simulink model "Control_test"  (R2014b)
settings: Solver=FixedStepDiscrete  StartTime=0.0  StopTime=Inf  FixedStep=0.001  RelTol=1e-3
PostLoadFcn:
  | , if any(exist('dsrtsu_mdlpostloadfcn', 'file') == [2, 3, 6]), try dsrtsu_mdlpostloadfcn('Execute', bdroot); catch fprintf('Error in PostLoadFcn (dsrtsu_mdlpostloadfcn) for model "%s":\n %s\n', bdroot, lasterr); end, end,
undefined symbols (not defined in the file or in its folder): dtLocal, slcm
libraries: rtican x163, simulink x14
(part 10 of 34)

== system Control_test/InputProcessing/CameraCanProcessing/Obstacle_Data_A_4 ==
  Bus Creator : BusCreator  Inputs=11
  Obstacle_Data_A_4 : rtican/RTICAN Receive (RX)   Reserved1=[]  Reserved2=[]  Reserved3=[]  Reserved4=[]  SfcnMessage=[]  Msg_Struct=[]  BoardTypeNo=[]  BoardNo=[]  ChannelNo=[]  Parameters=[]  DialogFcn=[]  UnitName=[]  Revision=[]  UnitValues=[]  DSProperties=struct('RTI',struct('Version',uint32(5),'BlockType',struct('isSLSource',uint8(1),'isSLSink',uint8(1),'isHWSource',uint8(0),'isHWSink',uint8(0),'isSetup',uint8(0),'isInline',uint8(1),'isNonInline',uint8(0),'isInterrupt',uint8(0),'isChannelwise',uint8(0)),'IOBoardType','RTICAN','UnitType','MESSAGE','Identifier','RX','DialogType','MSVC','BlockSet','RTICAN','SlaveProcessor','CAN'))  RTIBlockInterface=struct('OutputPortsWidth',int32([1 1 1 1 1 1 1 1 1 1 1]),'OutputPortsActive',[1 1 1 1 1 1 1 1 1 1 1],'OutputPortsName',{{'Alive_Counter_A_4','ObjectIdentifier_A_4','ObjectAge_A_4','AngleRate_A_4','AngleLeft_A_4','AngleRight_A_4','MotionStatus_A_4','ObjectLane_A_4','CIPV_A_4','ObstacleBrakeLights_A_4','BlinkerInfo_A_4'}},'OutputPortsDataType',{{'SS_DOUBLE','SS_DOUBLE','SS_DOUBLE','SS_DOUBLE','SS_DOUBLE','SS_DOUBLE','SS_DOUBLE','SS_DOUBLE','SS_DOUBLE','SS_DOUBLE','SS_DOUBLE'}},'OutputPortsLabel',{{'Alive_Counter_A_4','ObjectIdentifier_A_4','ObjectAge_A_4','AngleRate_A_4','AngleLeft_A_4','AngleRight_A_4','MotionStatus_A_4','ObjectLane_A_4','CIPV_A_4','ObstacleBrakeLights_A_4','BlinkerInfo_A_4'}},'OutputPortsLabelMode','ON','InputPortsWidth',int32(0),'InputPortsActive',0,'DialogFcn','rtican_message_interface_gui','BlockDisplay',{{'','center'}},'IconTransparency','on','ParameterTunableNames',{{}},'InitLevel',3,'BlockName',struct('Token',{{'Obstacle_Data_A_4'}}),'SampleTime',{{0.01}},'TriggerPort',{{'none'}},'EnablePort',{{'none'}})  RTIBlockParameters=struct('BoardTypeNo',{{1,'OFF',[]}},'BoardNo',{{1,'ON',[1 16]}},'ChannelNo',{{2,'ON',[1 2]}},'Parameters',{{struct('DataFileSupport',struct('DataFileSelectedMaster',1,'DataFileSelectedLocal',0,'DataFileName',['c:\users\mpc\dropbox\cpg_test_2014\t4_rfs_demo\hyundai car setup\rt2000_can_mod.dbc|c:\users\mpc\dropbox\cpg_test_2014\t4_rfs_demo\hyundai car setup\mobileye spec new\mobileye_mando_camera_ucb_v2.dbc|'],'DataFileDate',{{{['13-Nov-2012 16:29:35']},{['18-Sep-2013 10:55:24']}}},'SelectedFile',['<no file selected>'],'InterfaceFcn','rtican_dbc_file_parser'),'Options',struct('StatusSelected',0,'TimeSelected',0,'DeltaTimeSelected',0,'BytePortSelected',0,'MessageLengthSelected',0,'TriggerPort',struct('Selected',0,'TriggerType',0),'UserCoding',struct('Selected',0,'InterfaceFile','UserDecodingFile','FcnName','UserDecodeFcn','InportSelected',0,'InportWidth',1,'OutportSelected',0,'OutportWidth',1),'EnablePortSelected',0,'SignalOnPortnameSelected',1,'UseRXService',0),'Message',struct('MsgOnBlocknameSelected',1,'MsgName','Obstacle_Data_A_4','MsgIdFormat',0,'MsgId',1858,'MsgLength',8,'NumSignals',11,'SampleTime',0.01,'Signal',struct('SgnName',{'Alive_Counter_A_4','ObjectIdentifier_A_4','ObjectAge_A_4','AngleRate_A_4','AngleLeft_A_4','AngleRight_A_4','MotionStatus_A_4','ObjectLane_A_4','CIPV_A_4','ObstacleBrakeLights_A_4','BlinkerInfo_A_4'},'SgnStartBit',{0,2,8,16,28,40,52,56,60,61,62},'SgnLength',{2,6,8,12,12,12,4,4,1,1,2},'SgnType',{0,0,0,0,0,0,0,0,0,0,0},'ModeValue',{-1,-1,-1,-1,-1,-1,-1,-1,-1,-1,-1},'DataType',{0,0,0,0,0,0,0,0,0,0,0},'ByteLayout',{0,0,0,0,0,0,0,0,0,0,0},'Factor',{1,1,1,0.05,0.05,0.05,1,1,1,1,1},'Offset',{0,0,0,-100,-100,-100,0,0,0,0,0},'SgnComment',{{''},{''},{''},{''},{''},{''},{''},{''},{''},{''},{''}},'SgnUnit',{'','','','Deg','Deg','Deg','','','','',''},'Min',{0,0,0,0,0,0,0,0,0,0,0},'Max',{0,0,0,0,0,0,0,0,0,0,0},'SLDataType',{'SS_DOUBLE','SS_DOUBLE','SS_DOUBLE','SS_DOUBLE','SS_DOUBLE','SS_DOUBLE','SS_DOUBLE','SS_DOUBLE','SS_DOUBLE','SS_DOUBLE','SS_DOUBLE'}),'MsgIdNumFormat',1,'MsgComment',{{''}}),'Version',1.2,'general',struct('isFromLib',0)),'OFF',[]}},'GroupId',{{struct('Group',{{'RTICAN'}},'No',2,'Behavior',{{'NAMECHANGE'}},'BlockType',{{'SINK'}},'NameChangeFlag',0),'OFF',[]}},'SFcnRTICANMessage',{{struct('MsgType','RX','SFcnPortType','Scalar','MsgName','Obstacle_Data_A_4','MsgIdFormat','STD','MsgId',1858,'MsgLength',8,'NumSignals',11,'SampleTime',0.01,'Signal',struct('SgnName',{'Alive_Counter_A_4','ObjectIdentifier_A_4','ObjectAge_A_4','AngleRate_A_4','AngleLeft_A_4','AngleRight_A_4','MotionStatus_A_4','ObjectLane_A_4','CIPV_A_4','ObstacleBrakeLights_A_4','BlinkerInfo_A_4'},'SgnStartBit',{0,2,8,16,28,40,52,56,60,61,62},'SgnLength',{2,6,8,12,12,12,4,4,1,1,2},'SgnType',{'standard','standard','standard','standard','standard','standard','standard','standard','standard','standard','standard'},'ModeValue',{-1,-1,-1,-1,-1,-1,-1,-1,-1,-1,-1},'DataType',{['unsigned int'],['unsigned int'],['unsigned int'],['unsigned int'],['unsigned int'],['unsigned int'],['unsigned int'],['unsigned int'],['unsigned int'],['unsigned int'],['unsigned int']},'ByteLayout',{['little endian'],['little endian'],['little endian'],['little endian'],['little endian'],['little endian'],['little endian'],['little endian'],['little endian'],['little endian'],['little endian']},'Factor',{1,1,1,0.05,0.05,0.05,1,1,1,1,1},'Offset',{0,0,0,-100,-100,-100,0,0,0,0,0},'SLDataType',{'SS_DOUBLE','SS_DOUBLE','SS_DOUBLE','SS_DOUBLE','SS_DOUBLE','SS_DOUBLE','SS_DOUBLE','SS_DOUBLE','SS_DOUBLE','SS_DOUBLE','SS_DOUBLE'}),'StatusSelected','no','TimeSelected','no','DeltaTimeSelected','no','BytePortSelected','no','MessageLengthSelected','no','TriggerPort',struct('Selected','no','TriggerType',0),'UserCoding',struct('Selected','no','InterfaceFile','UserDecodingFile','FcnName','UserDecodeFcn','InportSelected','no','InportWidth',1,'OutportSelected','no','OutportWidth',1),'EnablePortSelected','no','UseRXService','no','BoardType','DS1','BoardNo',1,'ControllerNo',2),'OFF',[]}},'TLCFileName',{{'rtican_rx_message','OFF',[]}})  RTISFcnParameters=struct('SFcnRTICANMessage','struct','TLCFileName','char')  RTIBlockParaDefault=struct('BoardTypeNo',4302,'BoardNo',1,'ChannelNo',1,'Parameters',struct('DataFileSupport',struct('DataFileSelectedMaster',0,'DataFileSelectedLocal',0,'DataFileName','','DataFileDate','','SelectedFile',['<no file selected>']),'Options',struct('StatusSelected',1,'TimeSelected',1,'DeltaTimeSelected',1,'BytePortSelected',0,'MessageLengthSelected',0,'TriggerPort',struct('Selected',0,'TriggerType','rising'),'UserCoding',struct('Selected',0,'InterfaceFile','UserDecodingFile','FcnName','UserDecodeFcn','InportSelected',0,'InportWidth',1,'OutportSelected',0,'OutportWidth',1),'EnablePortSelected',0,'SignalOnPortnameSelected',1,'UseRXService',0),'Message',struct('MsgOnBlocknameSelected',0,'MsgName',['RX Message'],'MsgIdFormat',0,'MsgId',100,'MsgLength',8,'NumSignals',1,'SampleTime',-1,'Signal',struct('SgnName',['RX signal'],'SgnStartBit',0,'SgnLength',8,'SgnType',0,'ModeValue',-1,'DataType',0,'SLDataType','SS_DOUBLE','ByteLayout',0,'Factor',1,'Offset',0,'Min',0,'Max',255,'SgnComment',{{}},'SgnUnit',''),'MsgIdNumFormat',0,'MsgComment',{{''}}),'Version',1.2,'general',struct('isFromLib',1)),'GroupId',struct('Group',{{'RTICAN'}},'No',1,'Behavior',{{'NAMECHANGE'}},'BlockType',{{'SINK'}},'NameChangeFlag',0),'SFcnRTICANMessage',struct('MsgType','RX','MsgName',['RX Message'],'MsgIdFormat','STD','MsgId',100,'MsgLength',8,'NumSignals',1,'SampleTime',-1,'Signal',struct('SgnName',['RX signal'],'SgnStartBit',0,'SgnLength',8,'SgnType','standard','ModeValue',-1,'DataType',['unsigned int'],'ByteLayout',['little endian'],'SLDataType','SS_DOUBLE','Factor',1,'Offset',0),'StatusSelected','yes','TimeSelected','yes','DeltaTimeSelected','yes','BytePortSelected','no','MessageLengthSelected','no','EnablePortSelected','no','UserCoding',struct('Selected','no','InterfaceFile','UserDecodingFile','FcnName','UserDecodeFcn','InportSelected','no','InportWidth',1,'OutportSelected','no','OutportWidth',1),'TriggerPort',struct('Selected','no','TriggerType','rising'),'UseRXService','no','BoardType','DS4302','BoardNo',1,'ControllerNo',1,'SFcnPortType','Scalar'),'TLCFileName','rtican_rx_message')
      settings: AttributesFormatString=Group Id: RTICAN2\n
  Obstacle_Data_A_4_CAN : Outport
  wires:
  Bus Creator/1 -> Obstacle_Data_A_4_CAN/1
  Obstacle_Data_A_4/1 -> Bus Creator/1  "Alive_Counter_A_4"
  Obstacle_Data_A_4/2 -> Bus Creator/2  "ObjectIdentifier_A_4"
  Obstacle_Data_A_4/3 -> Bus Creator/3  "ObjectAge_A_4"
  Obstacle_Data_A_4/4 -> Bus Creator/4  "AngleRate_A_4"
  Obstacle_Data_A_4/5 -> Bus Creator/5  "AngleLeft_A_4"
  Obstacle_Data_A_4/6 -> Bus Creator/6  "AngleRight_A_4"
  Obstacle_Data_A_4/7 -> Bus Creator/7  "MotionStatus_A_4"
  Obstacle_Data_A_4/8 -> Bus Creator/8  "ObjectLane_A_4"
  Obstacle_Data_A_4/9 -> Bus Creator/9  "CIPV_A_4"
  Obstacle_Data_A_4/10 -> Bus Creator/10  "ObstacleBrakeLights_A_4"
  Obstacle_Data_A_4/11 -> Bus Creator/11  "BlinkerInfo_A_4"

== system Control_test/InputProcessing/CameraCanProcessing/Obstacle_Data_A_5 ==
  Bus Creator : BusCreator  Inputs=11
  Obstacle_Data_A_5 : rtican/RTICAN Receive (RX)   Reserved1=[]  Reserved2=[]  Reserved3=[]  Reserved4=[]  SfcnMessage=[]  Msg_Struct=[]  BoardTypeNo=[]  BoardNo=[]  ChannelNo=[]  Parameters=[]  DialogFcn=[]  UnitName=[]  Revision=[]  UnitValues=[]  DSProperties=struct('RTI',struct('Version',uint32(5),'BlockType',struct('isSLSource',uint8(1),'isSLSink',uint8(1),'isHWSource',uint8(0),'isHWSink',uint8(0),'isSetup',uint8(0),'isInline',uint8(1),'isNonInline',uint8(0),'isInterrupt',uint8(0),'isChannelwise',uint8(0)),'IOBoardType','RTICAN','UnitType','MESSAGE','Identifier','RX','DialogType','MSVC','BlockSet','RTICAN','SlaveProcessor','CAN'))  RTIBlockInterface=struct('OutputPortsWidth',int32([1 1 1 1 1 1 1 1 1 1 1]),'OutputPortsActive',[1 1 1 1 1 1 1 1 1 1 1],'OutputPortsName',{{'Alive_Counter_A_5','ObjectIdentifier_A_5','ObjectAge_A_5','AngleRate_A_5','AngleLeft_A_5','AngleRight_A_5','MotionStatus_A_5','ObjectLane_A_5','CIPV_A_5','ObstacleBrakeLights_A_5','BlinkerInfo_A_5'}},'OutputPortsDataType',{{'SS_DOUBLE','SS_DOUBLE','SS_DOUBLE','SS_DOUBLE','SS_DOUBLE','SS_DOUBLE','SS_DOUBLE','SS_DOUBLE','SS_DOUBLE','SS_DOUBLE','SS_DOUBLE'}},'OutputPortsLabel',{{'Alive_Counter_A_5','ObjectIdentifier_A_5','ObjectAge_A_5','AngleRate_A_5','AngleLeft_A_5','AngleRight_A_5','MotionStatus_A_5','ObjectLane_A_5','CIPV_A_5','ObstacleBrakeLights_A_5','BlinkerInfo_A_5'}},'OutputPortsLabelMode','ON','InputPortsWidth',int32(0),'InputPortsActive',0,'DialogFcn','rtican_message_interface_gui','BlockDisplay',{{'','center'}},'IconTransparency','on','ParameterTunableNames',{{}},'InitLevel',3,'BlockName',struct('Token',{{'Obstacle_Data_A_5'}}),'SampleTime',{{0.01}},'TriggerPort',{{'none'}},'EnablePort',{{'none'}})  RTIBlockParameters=struct('BoardTypeNo',{{1,'OFF',[]}},'BoardNo',{{1,'ON',[1 16]}},'ChannelNo',{{2,'ON',[1 2]}},'Parameters',{{struct('DataFileSupport',struct('DataFileSelectedMaster',1,'DataFileSelectedLocal',1,'DataFileName',['c:\users\mpc\desktop\hyundai car setup\rt2000_can_mod.dbc|c:\users\mpc\desktop\hyundai car setup\mobileye spec new\mobileye_mando_camera_ucb_v2.dbc|'],'DataFileDate',['18-Sep-2013 17:55:24'],'SelectedFile','..\..\dbcfiles\mobileye_mando_camera_ucb_v2.dbc','InterfaceFcn','rtican_dbc_file_parser'),'Options',struct('StatusSelected',0,'TimeSelected',0,'DeltaTimeSelected',0,'BytePortSelected',0,'MessageLengthSelected',0,'TriggerPort',struct('Selected',0,'TriggerType',0),'UserCoding',struct('Selected',0,'InterfaceFile','UserDecodingFile','FcnName','UserDecodeFcn','InportSelected',0,'InportWidth',1,'OutportSelected',0,'OutportWidth',1),'EnablePortSelected',0,'SignalOnPortnameSelected',1,'UseRXService',0),'Message',struct('MsgOnBlocknameSelected',1,'MsgName','Obstacle_Data_A_5','MsgIdFormat',0,'MsgId',1861,'MsgLength',8,'NumSignals',11,'SampleTime',0.01,'Signal',struct('SgnName',{'Alive_Counter_A_5','ObjectIdentifier_A_5','ObjectAge_A_5','AngleRate_A_5','AngleLeft_A_5','AngleRight_A_5','MotionStatus_A_5','ObjectLane_A_5','CIPV_A_5','ObstacleBrakeLights_A_5','BlinkerInfo_A_5'},'SgnStartBit',{0,2,8,16,28,40,52,56,60,61,62},'SgnLength',{2,6,8,12,12,12,4,4,1,1,2},'ByteLayout',{0,0,0,0,0,0,0,0,0,0,0},'Factor',{1,1,1,0.05,0.05,0.05,1,1,1,1,1},'Offset',{0,0,0,-100,-100,-100,0,0,0,0,0},'SgnComment',{'','','','','','','','','','',''},'SgnUnit',{'','','','Deg','Deg','Deg','','','','',''},'Min',{0,0,0,0,0,0,0,0,0,0,0},'Max',{0,0,0,0,0,0,0,0,0,0,0},'SgnType',{0,0,0,0,0,0,0,0,0,0,0},'SLDataType',{'SS_DOUBLE','SS_DOUBLE','SS_DOUBLE','SS_DOUBLE','SS_DOUBLE','SS_DOUBLE','SS_DOUBLE','SS_DOUBLE','SS_DOUBLE','SS_DOUBLE','SS_DOUBLE'},'DataType',{0,0,0,0,0,0,0,0,0,0,0},'ModeValue',{-1,-1,-1,-1,-1,-1,-1,-1,-1,-1,-1}),'MsgIdNumFormat',0,'MsgComment',{{''}}),'Version',1.2,'general',struct('isFromLib',0)),'OFF',[]}},'GroupId',{{struct('Group',{{'RTICAN'}},'No',2,'Behavior',{{'NAMECHANGE'}},'BlockType',{{'SINK'}},'NameChangeFlag',0),'OFF',[]}},'SFcnRTICANMessage',{{struct('MsgType','RX','SFcnPortType','Scalar','MsgName','Obstacle_Data_A_5','MsgIdFormat','STD','MsgId',1861,'MsgLength',8,'NumSignals',11,'SampleTime',0.01,'Signal',struct('SgnName',{'Alive_Counter_A_5','ObjectIdentifier_A_5','ObjectAge_A_5','AngleRate_A_5','AngleLeft_A_5','AngleRight_A_5','MotionStatus_A_5','ObjectLane_A_5','CIPV_A_5','ObstacleBrakeLights_A_5','BlinkerInfo_A_5'},'SgnStartBit',{0,2,8,16,28,40,52,56,60,61,62},'SgnLength',{2,6,8,12,12,12,4,4,1,1,2},'ByteLayout',{['little endian'],['little endian'],['little endian'],['little endian'],['little endian'],['little endian'],['little endian'],['little endian'],['little endian'],['little endian'],['little endian']},'Factor',{1,1,1,0.05,0.05,0.05,1,1,1,1,1},'Offset',{0,0,0,-100,-100,-100,0,0,0,0,0},'SgnType',{'standard','standard','standard','standard','standard','standard','standard','standard','standard','standard','standard'},'SLDataType',{'SS_DOUBLE','SS_DOUBLE','SS_DOUBLE','SS_DOUBLE','SS_DOUBLE','SS_DOUBLE','SS_DOUBLE','SS_DOUBLE','SS_DOUBLE','SS_DOUBLE','SS_DOUBLE'},'DataType',{['unsigned int'],['unsigned int'],['unsigned int'],['unsigned int'],['unsigned int'],['unsigned int'],['unsigned int'],['unsigned int'],['unsigned int'],['unsigned int'],['unsigned int']},'ModeValue',{-1,-1,-1,-1,-1,-1,-1,-1,-1,-1,-1}),'StatusSelected','no','TimeSelected','no','DeltaTimeSelected','no','BytePortSelected','no','MessageLengthSelected','no','TriggerPort',struct('Selected','no','TriggerType',0),'UserCoding',struct('Selected','no','InterfaceFile','UserDecodingFile','FcnName','UserDecodeFcn','InportSelected','no','InportWidth',1,'OutportSelected','no','OutportWidth',1),'EnablePortSelected','no','UseRXService','no','BoardType','DS1','BoardNo',1,'ControllerNo',2),'OFF',[]}},'TLCFileName',{{'rtican_rx_message','OFF',[]}})  RTISFcnParameters=struct('SFcnRTICANMessage','struct','TLCFileName','char')  RTIBlockParaDefault=struct('BoardTypeNo',4302,'BoardNo',1,'ChannelNo',1,'Parameters',struct('DataFileSupport',struct('DataFileSelectedMaster',0,'DataFileSelectedLocal',0,'DataFileName','','DataFileDate','','SelectedFile',['<no file selected>']),'Options',struct('StatusSelected',1,'TimeSelected',1,'DeltaTimeSelected',1,'BytePortSelected',0,'MessageLengthSelected',0,'TriggerPort',struct('Selected',0,'TriggerType','rising'),'UserCoding',struct('Selected',0,'InterfaceFile','UserDecodingFile','FcnName','UserDecodeFcn','InportSelected',0,'InportWidth',1,'OutportSelected',0,'OutportWidth',1),'EnablePortSelected',0,'SignalOnPortnameSelected',1,'UseRXService',0),'Message',struct('MsgOnBlocknameSelected',0,'MsgName',['RX Message'],'MsgIdFormat',0,'MsgId',100,'MsgLength',8,'NumSignals',1,'SampleTime',-1,'Signal',struct('SgnName',['RX signal'],'SgnStartBit',0,'SgnLength',8,'SgnType',0,'ModeValue',-1,'DataType',0,'SLDataType','SS_DOUBLE','ByteLayout',0,'Factor',1,'Offset',0,'Min',0,'Max',255,'SgnComment',{{}},'SgnUnit',''),'MsgIdNumFormat',0,'MsgComment',{{''}}),'Version',1.2,'general',struct('isFromLib',1)),'GroupId',struct('Group',{{'RTICAN'}},'No',1,'Behavior',{{'NAMECHANGE'}},'BlockType',{{'SINK'}},'NameChangeFlag',0),'SFcnRTICANMessage',struct('MsgType','RX','MsgName',['RX Message'],'MsgIdFormat','STD','MsgId',100,'MsgLength',8,'NumSignals',1,'SampleTime',-1,'Signal',struct('SgnName',['RX signal'],'SgnStartBit',0,'SgnLength',8,'SgnType','standard','ModeValue',-1,'DataType',['unsigned int'],'ByteLayout',['little endian'],'SLDataType','SS_DOUBLE','Factor',1,'Offset',0),'StatusSelected','yes','TimeSelected','yes','DeltaTimeSelected','yes','BytePortSelected','no','MessageLengthSelected','no','EnablePortSelected','no','UserCoding',struct('Selected','no','InterfaceFile','UserDecodingFile','FcnName','UserDecodeFcn','InportSelected','no','InportWidth',1,'OutportSelected','no','OutportWidth',1),'TriggerPort',struct('Selected','no','TriggerType','rising'),'UseRXService','no','BoardType','DS4302','BoardNo',1,'ControllerNo',1,'SFcnPortType','Scalar'),'TLCFileName','rtican_rx_message')
      settings: AttributesFormatString=Group Id: RTICAN2\n
  Obstacle_Data_A_5_CAN : Outport
  wires:
  Bus Creator/1 -> Obstacle_Data_A_5_CAN/1
  Obstacle_Data_A_5/1 -> Bus Creator/1  "Alive_Counter_A_5"
  Obstacle_Data_A_5/2 -> Bus Creator/2  "ObjectIdentifier_A_5"
  Obstacle_Data_A_5/3 -> Bus Creator/3  "ObjectAge_A_5"
  Obstacle_Data_A_5/4 -> Bus Creator/4  "AngleRate_A_5"
  Obstacle_Data_A_5/5 -> Bus Creator/5  "AngleLeft_A_5"
  Obstacle_Data_A_5/6 -> Bus Creator/6  "AngleRight_A_5"
  Obstacle_Data_A_5/7 -> Bus Creator/7  "MotionStatus_A_5"
  Obstacle_Data_A_5/8 -> Bus Creator/8  "ObjectLane_A_5"
  Obstacle_Data_A_5/9 -> Bus Creator/9  "CIPV_A_5"
  Obstacle_Data_A_5/10 -> Bus Creator/10  "ObstacleBrakeLights_A_5"
  Obstacle_Data_A_5/11 -> Bus Creator/11  "BlinkerInfo_A_5"

== system Control_test/InputProcessing/CameraCanProcessing/Obstacle_Data_A_6 ==
  Bus Creator : BusCreator  Inputs=11
  Obstacle_Data_A_6 : rtican/RTICAN Receive (RX)   Reserved1=[]  Reserved2=[]  Reserved3=[]  Reserved4=[]  SfcnMessage=[]  Msg_Struct=[]  BoardTypeNo=[]  BoardNo=[]  ChannelNo=[]  Parameters=[]  DialogFcn=[]  UnitName=[]  Revision=[]  UnitValues=[]  DSProperties=struct('RTI',struct('Version',uint32(5),'BlockType',struct('isSLSource',uint8(1),'isSLSink',uint8(1),'isHWSource',uint8(0),'isHWSink',uint8(0),'isSetup',uint8(0),'isInline',uint8(1),'isNonInline',uint8(0),'isInterrupt',uint8(0),'isChannelwise',uint8(0)),'IOBoardType','RTICAN','UnitType','MESSAGE','Identifier','RX','DialogType','MSVC','BlockSet','RTICAN','SlaveProcessor','CAN'))  RTIBlockInterface=struct('OutputPortsWidth',int32([1 1 1 1 1 1 1 1 1 1 1]),'OutputPortsActive',[1 1 1 1 1 1 1 1 1 1 1],'OutputPortsName',{{'Alive_Counter_A_6','ObjectIdentifier_A_6','ObjectAge_A_6','AngleRate_A_6','AngleLeft_A_6','AngleRight_A_6','MotionStatus_A_6','ObjectLane_A_6','CIPV_A_6','ObstacleBrakeLights_A_6','BlinkerInfo_A_6'}},'OutputPortsDataType',{{'SS_DOUBLE','SS_DOUBLE','SS_DOUBLE','SS_DOUBLE','SS_DOUBLE','SS_DOUBLE','SS_DOUBLE','SS_DOUBLE','SS_DOUBLE','SS_DOUBLE','SS_DOUBLE'}},'OutputPortsLabel',{{'Alive_Counter_A_6','ObjectIdentifier_A_6','ObjectAge_A_6','AngleRate_A_6','AngleLeft_A_6','AngleRight_A_6','MotionStatus_A_6','ObjectLane_A_6','CIPV_A_6','ObstacleBrakeLights_A_6','BlinkerInfo_A_6'}},'OutputPortsLabelMode','ON','InputPortsWidth',int32(0),'InputPortsActive',0,'DialogFcn','rtican_message_interface_gui','BlockDisplay',{{'','center'}},'IconTransparency','on','ParameterTunableNames',{{}},'InitLevel',3,'BlockName',struct('Token',{{'Obstacle_Data_A_6'}}),'SampleTime',{{0.01}},'TriggerPort',{{'none'}},'EnablePort',{{'none'}})  RTIBlockParameters=struct('BoardTypeNo',{{1,'OFF',[]}},'BoardNo',{{1,'ON',[1 16]}},'ChannelNo',{{2,'ON',[1 2]}},'Parameters',{{struct('DataFileSupport',struct('DataFileSelectedMaster',1,'DataFileSelectedLocal',1,'DataFileName',['c:\users\mpc\desktop\hyundai car setup\rt2000_can_mod.dbc|c:\users\mpc\desktop\hyundai car setup\mobileye spec new\mobileye_mando_camera_ucb_v2.dbc|'],'DataFileDate',['18-Sep-2013 17:55:24'],'SelectedFile','..\..\dbcfiles\mobileye_mando_camera_ucb_v2.dbc','InterfaceFcn','rtican_dbc_file_parser'),'Options',struct('StatusSelected',0,'TimeSelected',0,'DeltaTimeSelected',0,'BytePortSelected',0,'MessageLengthSelected',0,'TriggerPort',struct('Selected',0,'TriggerType',0),'UserCoding',struct('Selected',0,'InterfaceFile','UserDecodingFile','FcnName','UserDecodeFcn','InportSelected',0,'InportWidth',1,'OutportSelected',0,'OutportWidth',1),'EnablePortSelected',0,'SignalOnPortnameSelected',1,'UseRXService',0),'Message',struct('MsgOnBlocknameSelected',1,'MsgName','Obstacle_Data_A_6','MsgIdFormat',0,'MsgId',1864,'MsgLength',8,'NumSignals',11,'SampleTime',0.01,'Signal',struct('SgnName',{'Alive_Counter_A_6','ObjectIdentifier_A_6','ObjectAge_A_6','AngleRate_A_6','AngleLeft_A_6','AngleRight_A_6','MotionStatus_A_6','ObjectLane_A_6','CIPV_A_6','ObstacleBrakeLights_A_6','BlinkerInfo_A_6'},'SgnStartBit',{0,2,8,16,28,40,52,56,60,61,62},'SgnLength',{2,6,8,12,12,12,4,4,1,1,2},'ByteLayout',{0,0,0,0,0,0,0,0,0,0,0},'Factor',{1,1,1,0.05,0.05,0.05,1,1,1,1,1},'Offset',{0,0,0,-100,-100,-100,0,0,0,0,0},'SgnComment',{'','','','','','','','','','',''},'SgnUnit',{'','','','Deg','Deg','Deg','','','','',''},'Min',{0,0,0,0,0,0,0,0,0,0,0},'Max',{0,0,0,0,0,0,0,0,0,0,0},'SgnType',{0,0,0,0,0,0,0,0,0,0,0},'SLDataType',{'SS_DOUBLE','SS_DOUBLE','SS_DOUBLE','SS_DOUBLE','SS_DOUBLE','SS_DOUBLE','SS_DOUBLE','SS_DOUBLE','SS_DOUBLE','SS_DOUBLE','SS_DOUBLE'},'DataType',{0,0,0,0,0,0,0,0,0,0,0},'ModeValue',{-1,-1,-1,-1,-1,-1,-1,-1,-1,-1,-1}),'MsgIdNumFormat',0,'MsgComment',{{''}}),'Version',1.2,'general',struct('isFromLib',0)),'OFF',[]}},'GroupId',{{struct('Group',{{'RTICAN'}},'No',2,'Behavior',{{'NAMECHANGE'}},'BlockType',{{'SINK'}},'NameChangeFlag',0),'OFF',[]}},'SFcnRTICANMessage',{{struct('MsgType','RX','SFcnPortType','Scalar','MsgName','Obstacle_Data_A_6','MsgIdFormat','STD','MsgId',1864,'MsgLength',8,'NumSignals',11,'SampleTime',0.01,'Signal',struct('SgnName',{'Alive_Counter_A_6','ObjectIdentifier_A_6','ObjectAge_A_6','AngleRate_A_6','AngleLeft_A_6','AngleRight_A_6','MotionStatus_A_6','ObjectLane_A_6','CIPV_A_6','ObstacleBrakeLights_A_6','BlinkerInfo_A_6'},'SgnStartBit',{0,2,8,16,28,40,52,56,60,61,62},'SgnLength',{2,6,8,12,12,12,4,4,1,1,2},'ByteLayout',{['little endian'],['little endian'],['little endian'],['little endian'],['little endian'],['little endian'],['little endian'],['little endian'],['little endian'],['little endian'],['little endian']},'Factor',{1,1,1,0.05,0.05,0.05,1,1,1,1,1},'Offset',{0,0,0,-100,-100,-100,0,0,0,0,0},'SgnType',{'standard','standard','standard','standard','standard','standard','standard','standard','standard','standard','standard'},'SLDataType',{'SS_DOUBLE','SS_DOUBLE','SS_DOUBLE','SS_DOUBLE','SS_DOUBLE','SS_DOUBLE','SS_DOUBLE','SS_DOUBLE','SS_DOUBLE','SS_DOUBLE','SS_DOUBLE'},'DataType',{['unsigned int'],['unsigned int'],['unsigned int'],['unsigned int'],['unsigned int'],['unsigned int'],['unsigned int'],['unsigned int'],['unsigned int'],['unsigned int'],['unsigned int']},'ModeValue',{-1,-1,-1,-1,-1,-1,-1,-1,-1,-1,-1}),'StatusSelected','no','TimeSelected','no','DeltaTimeSelected','no','BytePortSelected','no','MessageLengthSelected','no','TriggerPort',struct('Selected','no','TriggerType',0),'UserCoding',struct('Selected','no','InterfaceFile','UserDecodingFile','FcnName','UserDecodeFcn','InportSelected','no','InportWidth',1,'OutportSelected','no','OutportWidth',1),'EnablePortSelected','no','UseRXService','no','BoardType','DS1','BoardNo',1,'ControllerNo',2),'OFF',[]}},'TLCFileName',{{'rtican_rx_message','OFF',[]}})  RTISFcnParameters=struct('SFcnRTICANMessage','struct','TLCFileName','char')  RTIBlockParaDefault=struct('BoardTypeNo',4302,'BoardNo',1,'ChannelNo',1,'Parameters',struct('DataFileSupport',struct('DataFileSelectedMaster',0,'DataFileSelectedLocal',0,'DataFileName','','DataFileDate','','SelectedFile',['<no file selected>']),'Options',struct('StatusSelected',1,'TimeSelected',1,'DeltaTimeSelected',1,'BytePortSelected',0,'MessageLengthSelected',0,'TriggerPort',struct('Selected',0,'TriggerType','rising'),'UserCoding',struct('Selected',0,'InterfaceFile','UserDecodingFile','FcnName','UserDecodeFcn','InportSelected',0,'InportWidth',1,'OutportSelected',0,'OutportWidth',1),'EnablePortSelected',0,'SignalOnPortnameSelected',1,'UseRXService',0),'Message',struct('MsgOnBlocknameSelected',0,'MsgName',['RX Message'],'MsgIdFormat',0,'MsgId',100,'MsgLength',8,'NumSignals',1,'SampleTime',-1,'Signal',struct('SgnName',['RX signal'],'SgnStartBit',0,'SgnLength',8,'SgnType',0,'ModeValue',-1,'DataType',0,'SLDataType','SS_DOUBLE','ByteLayout',0,'Factor',1,'Offset',0,'Min',0,'Max',255,'SgnComment',{{}},'SgnUnit',''),'MsgIdNumFormat',0,'MsgComment',{{''}}),'Version',1.2,'general',struct('isFromLib',1)),'GroupId',struct('Group',{{'RTICAN'}},'No',1,'Behavior',{{'NAMECHANGE'}},'BlockType',{{'SINK'}},'NameChangeFlag',0),'SFcnRTICANMessage',struct('MsgType','RX','MsgName',['RX Message'],'MsgIdFormat','STD','MsgId',100,'MsgLength',8,'NumSignals',1,'SampleTime',-1,'Signal',struct('SgnName',['RX signal'],'SgnStartBit',0,'SgnLength',8,'SgnType','standard','ModeValue',-1,'DataType',['unsigned int'],'ByteLayout',['little endian'],'SLDataType','SS_DOUBLE','Factor',1,'Offset',0),'StatusSelected','yes','TimeSelected','yes','DeltaTimeSelected','yes','BytePortSelected','no','MessageLengthSelected','no','EnablePortSelected','no','UserCoding',struct('Selected','no','InterfaceFile','UserDecodingFile','FcnName','UserDecodeFcn','InportSelected','no','InportWidth',1,'OutportSelected','no','OutportWidth',1),'TriggerPort',struct('Selected','no','TriggerType','rising'),'UseRXService','no','BoardType','DS4302','BoardNo',1,'ControllerNo',1,'SFcnPortType','Scalar'),'TLCFileName','rtican_rx_message')
      settings: AttributesFormatString=Group Id: RTICAN2\n
  Obstacle_Data_A_6_CAN : Outport
  wires:
  Bus Creator/1 -> Obstacle_Data_A_6_CAN/1
  Obstacle_Data_A_6/1 -> Bus Creator/1  "Alive_Counter_A_6"
  Obstacle_Data_A_6/2 -> Bus Creator/2  "ObjectIdentifier_A_6"
  Obstacle_Data_A_6/3 -> Bus Creator/3  "ObjectAge_A_6"
  Obstacle_Data_A_6/4 -> Bus Creator/4  "AngleRate_A_6"
  Obstacle_Data_A_6/5 -> Bus Creator/5  "AngleLeft_A_6"
  Obstacle_Data_A_6/6 -> Bus Creator/6  "AngleRight_A_6"
  Obstacle_Data_A_6/7 -> Bus Creator/7  "MotionStatus_A_6"
  Obstacle_Data_A_6/8 -> Bus Creator/8  "ObjectLane_A_6"
  Obstacle_Data_A_6/9 -> Bus Creator/9  "CIPV_A_6"
  Obstacle_Data_A_6/10 -> Bus Creator/10  "ObstacleBrakeLights_A_6"
  Obstacle_Data_A_6/11 -> Bus Creator/11  "BlinkerInfo_A_6"

== system Control_test/InputProcessing/CameraCanProcessing/Obstacle_Data_A_7 ==
  Bus Creator : BusCreator  Inputs=11
  Obstacle_Data_A_7 : rtican/RTICAN Receive (RX)   Reserved1=[]  Reserved2=[]  Reserved3=[]  Reserved4=[]  SfcnMessage=[]  Msg_Struct=[]  BoardTypeNo=[]  BoardNo=[]  ChannelNo=[]  Parameters=[]  DialogFcn=[]  UnitName=[]  Revision=[]  UnitValues=[]  DSProperties=struct('RTI',struct('Version',uint32(5),'BlockType',struct('isSLSource',uint8(1),'isSLSink',uint8(1),'isHWSource',uint8(0),'isHWSink',uint8(0),'isSetup',uint8(0),'isInline',uint8(1),'isNonInline',uint8(0),'isInterrupt',uint8(0),'isChannelwise',uint8(0)),'IOBoardType','RTICAN','UnitType','MESSAGE','Identifier','RX','DialogType','MSVC','BlockSet','RTICAN','SlaveProcessor','CAN'))  RTIBlockInterface=struct('OutputPortsWidth',int32([1 1 1 1 1 1 1 1 1 1 1]),'OutputPortsActive',[1 1 1 1 1 1 1 1 1 1 1],'OutputPortsName',{{'Alive_Counter_A_7','ObjectIdentifier_A_7','ObjectAge_A_7','AngleRate_A_7','AngleLeft_A_7','AngleRight_A_7','MotionStatus_A_7','ObjectLane_A_7','CIPV_A_7','ObstacleBrakeLights_A_7','BlinkerInfo_A_7'}},'OutputPortsDataType',{{'SS_DOUBLE','SS_DOUBLE','SS_DOUBLE','SS_DOUBLE','SS_DOUBLE','SS_DOUBLE','SS_DOUBLE','SS_DOUBLE','SS_DOUBLE','SS_DOUBLE','SS_DOUBLE'}},'OutputPortsLabel',{{'Alive_Counter_A_7','ObjectIdentifier_A_7','ObjectAge_A_7','AngleRate_A_7','AngleLeft_A_7','AngleRight_A_7','MotionStatus_A_7','ObjectLane_A_7','CIPV_A_7','ObstacleBrakeLights_A_7','BlinkerInfo_A_7'}},'OutputPortsLabelMode','ON','InputPortsWidth',int32(0),'InputPortsActive',0,'DialogFcn','rtican_message_interface_gui','BlockDisplay',{{'','center'}},'IconTransparency','on','ParameterTunableNames',{{}},'InitLevel',3,'BlockName',struct('Token',{{'Obstacle_Data_A_7'}}),'SampleTime',{{0.01}},'TriggerPort',{{'none'}},'EnablePort',{{'none'}})  RTIBlockParameters=struct('BoardTypeNo',{{1,'OFF',[]}},'BoardNo',{{1,'ON',[1 16]}},'ChannelNo',{{2,'ON',[1 2]}},'Parameters',{{struct('DataFileSupport',struct('DataFileSelectedMaster',1,'DataFileSelectedLocal',1,'DataFileName',['c:\users\mpc\desktop\hyundai car setup\rt2000_can_mod.dbc|c:\users\mpc\desktop\hyundai car setup\mobileye spec new\mobileye_mando_camera_ucb_v2.dbc|'],'DataFileDate',['18-Sep-2013 17:55:24'],'SelectedFile','..\..\dbcfiles\mobileye_mando_camera_ucb_v2.dbc','InterfaceFcn','rtican_dbc_file_parser'),'Options',struct('StatusSelected',0,'TimeSelected',0,'DeltaTimeSelected',0,'BytePortSelected',0,'MessageLengthSelected',0,'TriggerPort',struct('Selected',0,'TriggerType',0),'UserCoding',struct('Selected',0,'InterfaceFile','UserDecodingFile','FcnName','UserDecodeFcn','InportSelected',0,'InportWidth',1,'OutportSelected',0,'OutportWidth',1),'EnablePortSelected',0,'SignalOnPortnameSelected',1,'UseRXService',0),'Message',struct('MsgOnBlocknameSelected',1,'MsgName','Obstacle_Data_A_7','MsgIdFormat',0,'MsgId',1867,'MsgLength',8,'NumSignals',11,'SampleTime',0.01,'Signal',struct('SgnName',{'Alive_Counter_A_7','ObjectIdentifier_A_7','ObjectAge_A_7','AngleRate_A_7','AngleLeft_A_7','AngleRight_A_7','MotionStatus_A_7','ObjectLane_A_7','CIPV_A_7','ObstacleBrakeLights_A_7','BlinkerInfo_A_7'},'SgnStartBit',{0,2,8,16,28,40,52,56,60,61,62},'SgnLength',{2,6,8,12,12,12,4,4,1,1,2},'ByteLayout',{0,0,0,0,0,0,0,0,0,0,0},'Factor',{1,1,1,0.05,0.05,0.05,1,1,1,1,1},'Offset',{0,0,0,-100,-100,-100,0,0,0,0,0},'SgnComment',{'','','','','','','','','','',''},'SgnUnit',{'','','','Deg','Deg','Deg','','','','',''},'Min',{0,0,0,0,0,0,0,0,0,0,0},'Max',{0,0,0,0,0,0,0,0,0,0,0},'SgnType',{0,0,0,0,0,0,0,0,0,0,0},'SLDataType',{'SS_DOUBLE','SS_DOUBLE','SS_DOUBLE','SS_DOUBLE','SS_DOUBLE','SS_DOUBLE','SS_DOUBLE','SS_DOUBLE','SS_DOUBLE','SS_DOUBLE','SS_DOUBLE'},'DataType',{0,0,0,0,0,0,0,0,0,0,0},'ModeValue',{-1,-1,-1,-1,-1,-1,-1,-1,-1,-1,-1}),'MsgIdNumFormat',0,'MsgComment',{{''}}),'Version',1.2,'general',struct('isFromLib',0)),'OFF',[]}},'GroupId',{{struct('Group',{{'RTICAN'}},'No',2,'Behavior',{{'NAMECHANGE'}},'BlockType',{{'SINK'}},'NameChangeFlag',0),'OFF',[]}},'SFcnRTICANMessage',{{struct('MsgType','RX','SFcnPortType','Scalar','MsgName','Obstacle_Data_A_7','MsgIdFormat','STD','MsgId',1867,'MsgLength',8,'NumSignals',11,'SampleTime',0.01,'Signal',struct('SgnName',{'Alive_Counter_A_7','ObjectIdentifier_A_7','ObjectAge_A_7','AngleRate_A_7','AngleLeft_A_7','AngleRight_A_7','MotionStatus_A_7','ObjectLane_A_7','CIPV_A_7','ObstacleBrakeLights_A_7','BlinkerInfo_A_7'},'SgnStartBit',{0,2,8,16,28,40,52,56,60,61,62},'SgnLength',{2,6,8,12,12,12,4,4,1,1,2},'ByteLayout',{['little endian'],['little endian'],['little endian'],['little endian'],['little endian'],['little endian'],['little endian'],['little endian'],['little endian'],['little endian'],['little endian']},'Factor',{1,1,1,0.05,0.05,0.05,1,1,1,1,1},'Offset',{0,0,0,-100,-100,-100,0,0,0,0,0},'SgnType',{'standard','standard','standard','standard','standard','standard','standard','standard','standard','standard','standard'},'SLDataType',{'SS_DOUBLE','SS_DOUBLE','SS_DOUBLE','SS_DOUBLE','SS_DOUBLE','SS_DOUBLE','SS_DOUBLE','SS_DOUBLE','SS_DOUBLE','SS_DOUBLE','SS_DOUBLE'},'DataType',{['unsigned int'],['unsigned int'],['unsigned int'],['unsigned int'],['unsigned int'],['unsigned int'],['unsigned int'],['unsigned int'],['unsigned int'],['unsigned int'],['unsigned int']},'ModeValue',{-1,-1,-1,-1,-1,-1,-1,-1,-1,-1,-1}),'StatusSelected','no','TimeSelected','no','DeltaTimeSelected','no','BytePortSelected','no','MessageLengthSelected','no','TriggerPort',struct('Selected','no','TriggerType',0),'UserCoding',struct('Selected','no','InterfaceFile','UserDecodingFile','FcnName','UserDecodeFcn','InportSelected','no','InportWidth',1,'OutportSelected','no','OutportWidth',1),'EnablePortSelected','no','UseRXService','no','BoardType','DS1','BoardNo',1,'ControllerNo',2),'OFF',[]}},'TLCFileName',{{'rtican_rx_message','OFF',[]}})  RTISFcnParameters=struct('SFcnRTICANMessage','struct','TLCFileName','char')  RTIBlockParaDefault=struct('BoardTypeNo',4302,'BoardNo',1,'ChannelNo',1,'Parameters',struct('DataFileSupport',struct('DataFileSelectedMaster',0,'DataFileSelectedLocal',0,'DataFileName','','DataFileDate','','SelectedFile',['<no file selected>']),'Options',struct('StatusSelected',1,'TimeSelected',1,'DeltaTimeSelected',1,'BytePortSelected',0,'MessageLengthSelected',0,'TriggerPort',struct('Selected',0,'TriggerType','rising'),'UserCoding',struct('Selected',0,'InterfaceFile','UserDecodingFile','FcnName','UserDecodeFcn','InportSelected',0,'InportWidth',1,'OutportSelected',0,'OutportWidth',1),'EnablePortSelected',0,'SignalOnPortnameSelected',1,'UseRXService',0),'Message',struct('MsgOnBlocknameSelected',0,'MsgName',['RX Message'],'MsgIdFormat',0,'MsgId',100,'MsgLength',8,'NumSignals',1,'SampleTime',-1,'Signal',struct('SgnName',['RX signal'],'SgnStartBit',0,'SgnLength',8,'SgnType',0,'ModeValue',-1,'DataType',0,'SLDataType','SS_DOUBLE','ByteLayout',0,'Factor',1,'Offset',0,'Min',0,'Max',255,'SgnComment',{{}},'SgnUnit',''),'MsgIdNumFormat',0,'MsgComment',{{''}}),'Version',1.2,'general',struct('isFromLib',1)),'GroupId',struct('Group',{{'RTICAN'}},'No',1,'Behavior',{{'NAMECHANGE'}},'BlockType',{{'SINK'}},'NameChangeFlag',0),'SFcnRTICANMessage',struct('MsgType','RX','MsgName',['RX Message'],'MsgIdFormat','STD','MsgId',100,'MsgLength',8,'NumSignals',1,'SampleTime',-1,'Signal',struct('SgnName',['RX signal'],'SgnStartBit',0,'SgnLength',8,'SgnType','standard','ModeValue',-1,'DataType',['unsigned int'],'ByteLayout',['little endian'],'SLDataType','SS_DOUBLE','Factor',1,'Offset',0),'StatusSelected','yes','TimeSelected','yes','DeltaTimeSelected','yes','BytePortSelected','no','MessageLengthSelected','no','EnablePortSelected','no','UserCoding',struct('Selected','no','InterfaceFile','UserDecodingFile','FcnName','UserDecodeFcn','InportSelected','no','InportWidth',1,'OutportSelected','no','OutportWidth',1),'TriggerPort',struct('Selected','no','TriggerType','rising'),'UseRXService','no','BoardType','DS4302','BoardNo',1,'ControllerNo',1,'SFcnPortType','Scalar'),'TLCFileName','rtican_rx_message')
      settings: AttributesFormatString=Group Id: RTICAN2\n
  Obstacle_Data_A_7_CAN : Outport
  wires:
  Bus Creator/1 -> Obstacle_Data_A_7_CAN/1
  Obstacle_Data_A_7/1 -> Bus Creator/1  "Alive_Counter_A_7"
  Obstacle_Data_A_7/2 -> Bus Creator/2  "ObjectIdentifier_A_7"
  Obstacle_Data_A_7/3 -> Bus Creator/3  "ObjectAge_A_7"
  Obstacle_Data_A_7/4 -> Bus Creator/4  "AngleRate_A_7"
  Obstacle_Data_A_7/5 -> Bus Creator/5  "AngleLeft_A_7"
  Obstacle_Data_A_7/6 -> Bus Creator/6  "AngleRight_A_7"
  Obstacle_Data_A_7/7 -> Bus Creator/7  "MotionStatus_A_7"
  Obstacle_Data_A_7/8 -> Bus Creator/8  "ObjectLane_A_7"
  Obstacle_Data_A_7/9 -> Bus Creator/9  "CIPV_A_7"
  Obstacle_Data_A_7/10 -> Bus Creator/10  "ObstacleBrakeLights_A_7"
  Obstacle_Data_A_7/11 -> Bus Creator/11  "BlinkerInfo_A_7"

== system Control_test/InputProcessing/CameraCanProcessing/Obstacle_Data_A_8 ==
  Bus Creator : BusCreator  Inputs=11
  Obstacle_Data_A_8 : rtican/RTICAN Receive (RX)   Reserved1=[]  Reserved2=[]  Reserved3=[]  Reserved4=[]  SfcnMessage=[]  Msg_Struct=[]  BoardTypeNo=[]  BoardNo=[]  ChannelNo=[]  Parameters=[]  DialogFcn=[]  UnitName=[]  Revision=[]  UnitValues=[]  DSProperties=struct('RTI',struct('Version',uint32(5),'BlockType',struct('isSLSource',uint8(1),'isSLSink',uint8(1),'isHWSource',uint8(0),'isHWSink',uint8(0),'isSetup',uint8(0),'isInline',uint8(1),'isNonInline',uint8(0),'isInterrupt',uint8(0),'isChannelwise',uint8(0)),'IOBoardType','RTICAN','UnitType','MESSAGE','Identifier','RX','DialogType','MSVC','BlockSet','RTICAN','SlaveProcessor','CAN'))  RTIBlockInterface=struct('OutputPortsWidth',int32([1 1 1 1 1 1 1 1 1 1 1]),'OutputPortsActive',[1 1 1 1 1 1 1 1 1 1 1],'OutputPortsName',{{'Alive_Counter_A_8','ObjectIdentifier_A_8','ObjectAge_A_8','AngleRate_A_8','AngleLeft_A_8','AngleRight_A_8','MotionStatus_A_8','ObjectLane_A_8','CIPV_A_8','ObstacleBrakeLights_A_8','BlinkerInfo_A_8'}},'OutputPortsDataType',{{'SS_DOUBLE','SS_DOUBLE','SS_DOUBLE','SS_DOUBLE','SS_DOUBLE','SS_DOUBLE','SS_DOUBLE','SS_DOUBLE','SS_DOUBLE','SS_DOUBLE','SS_DOUBLE'}},'OutputPortsLabel',{{'Alive_Counter_A_8','ObjectIdentifier_A_8','ObjectAge_A_8','AngleRate_A_8','AngleLeft_A_8','AngleRight_A_8','MotionStatus_A_8','ObjectLane_A_8','CIPV_A_8','ObstacleBrakeLights_A_8','BlinkerInfo_A_8'}},'OutputPortsLabelMode','ON','InputPortsWidth',int32(0),'InputPortsActive',0,'DialogFcn','rtican_message_interface_gui','BlockDisplay',{{'','center'}},'IconTransparency','on','ParameterTunableNames',{{}},'InitLevel',3,'BlockName',struct('Token',{{'Obstacle_Data_A_8'}}),'SampleTime',{{0.01}},'TriggerPort',{{'none'}},'EnablePort',{{'none'}})  RTIBlockParameters=struct('BoardTypeNo',{{1,'OFF',[]}},'BoardNo',{{1,'ON',[1 16]}},'ChannelNo',{{2,'ON',[1 2]}},'Parameters',{{struct('DataFileSupport',struct('DataFileSelectedMaster',1,'DataFileSelectedLocal',1,'DataFileName',['c:\users\mpc\desktop\hyundai car setup\rt2000_can_mod.dbc|c:\users\mpc\desktop\hyundai car setup\mobileye spec new\mobileye_mando_camera_ucb_v2.dbc|'],'DataFileDate',['18-Sep-2013 17:55:24'],'SelectedFile','..\..\dbcfiles\mobileye_mando_camera_ucb_v2.dbc','InterfaceFcn','rtican_dbc_file_parser'),'Options',struct('StatusSelected',0,'TimeSelected',0,'DeltaTimeSelected',0,'BytePortSelected',0,'MessageLengthSelected',0,'TriggerPort',struct('Selected',0,'TriggerType',0),'UserCoding',struct('Selected',0,'InterfaceFile','UserDecodingFile','FcnName','UserDecodeFcn','InportSelected',0,'InportWidth',1,'OutportSelected',0,'OutportWidth',1),'EnablePortSelected',0,'SignalOnPortnameSelected',1,'UseRXService',0),'Message',struct('MsgOnBlocknameSelected',1,'MsgName','Obstacle_Data_A_8','MsgIdFormat',0,'MsgId',1870,'MsgLength',8,'NumSignals',11,'SampleTime',0.01,'Signal',struct('SgnName',{'Alive_Counter_A_8','ObjectIdentifier_A_8','ObjectAge_A_8','AngleRate_A_8','AngleLeft_A_8','AngleRight_A_8','MotionStatus_A_8','ObjectLane_A_8','CIPV_A_8','ObstacleBrakeLights_A_8','BlinkerInfo_A_8'},'SgnStartBit',{0,2,8,16,28,40,52,56,60,61,62},'SgnLength',{2,6,8,12,12,12,4,4,1,1,2},'ByteLayout',{0,0,0,0,0,0,0,0,0,0,0},'Factor',{1,1,1,0.05,0.05,0.05,1,1,1,1,1},'Offset',{0,0,0,-100,-100,-100,0,0,0,0,0},'SgnComment',{'','','','','','','','','','',''},'SgnUnit',{'','','','Deg','Deg','Deg','','','','',''},'Min',{0,0,0,0,0,0,0,0,0,0,0},'Max',{0,0,0,0,0,0,0,0,0,0,0},'SgnType',{0,0,0,0,0,0,0,0,0,0,0},'SLDataType',{'SS_DOUBLE','SS_DOUBLE','SS_DOUBLE','SS_DOUBLE','SS_DOUBLE','SS_DOUBLE','SS_DOUBLE','SS_DOUBLE','SS_DOUBLE','SS_DOUBLE','SS_DOUBLE'},'DataType',{0,0,0,0,0,0,0,0,0,0,0},'ModeValue',{-1,-1,-1,-1,-1,-1,-1,-1,-1,-1,-1}),'MsgIdNumFormat',0,'MsgComment',{{''}}),'Version',1.2,'general',struct('isFromLib',0)),'OFF',[]}},'GroupId',{{struct('Group',{{'RTICAN'}},'No',2,'Behavior',{{'NAMECHANGE'}},'BlockType',{{'SINK'}},'NameChangeFlag',0),'OFF',[]}},'SFcnRTICANMessage',{{struct('MsgType','RX','SFcnPortType','Scalar','MsgName','Obstacle_Data_A_8','MsgIdFormat','STD','MsgId',1870,'MsgLength',8,'NumSignals',11,'SampleTime',0.01,'Signal',struct('SgnName',{'Alive_Counter_A_8','ObjectIdentifier_A_8','ObjectAge_A_8','AngleRate_A_8','AngleLeft_A_8','AngleRight_A_8','MotionStatus_A_8','ObjectLane_A_8','CIPV_A_8','ObstacleBrakeLights_A_8','BlinkerInfo_A_8'},'SgnStartBit',{0,2,8,16,28,40,52,56,60,61,62},'SgnLength',{2,6,8,12,12,12,4,4,1,1,2},'ByteLayout',{['little endian'],['little endian'],['little endian'],['little endian'],['little endian'],['little endian'],['little endian'],['little endian'],['little endian'],['little endian'],['little endian']},'Factor',{1,1,1,0.05,0.05,0.05,1,1,1,1,1},'Offset',{0,0,0,-100,-100,-100,0,0,0,0,0},'SgnType',{'standard','standard','standard','standard','standard','standard','standard','standard','standard','standard','standard'},'SLDataType',{'SS_DOUBLE','SS_DOUBLE','SS_DOUBLE','SS_DOUBLE','SS_DOUBLE','SS_DOUBLE','SS_DOUBLE','SS_DOUBLE','SS_DOUBLE','SS_DOUBLE','SS_DOUBLE'},'DataType',{['unsigned int'],['unsigned int'],['unsigned int'],['unsigned int'],['unsigned int'],['unsigned int'],['unsigned int'],['unsigned int'],['unsigned int'],['unsigned int'],['unsigned int']},'ModeValue',{-1,-1,-1,-1,-1,-1,-1,-1,-1,-1,-1}),'StatusSelected','no','TimeSelected','no','DeltaTimeSelected','no','BytePortSelected','no','MessageLengthSelected','no','TriggerPort',struct('Selected','no','TriggerType',0),'UserCoding',struct('Selected','no','InterfaceFile','UserDecodingFile','FcnName','UserDecodeFcn','InportSelected','no','InportWidth',1,'OutportSelected','no','OutportWidth',1),'EnablePortSelected','no','UseRXService','no','BoardType','DS1','BoardNo',1,'ControllerNo',2),'OFF',[]}},'TLCFileName',{{'rtican_rx_message','OFF',[]}})  RTISFcnParameters=struct('SFcnRTICANMessage','struct','TLCFileName','char')  RTIBlockParaDefault=struct('BoardTypeNo',4302,'BoardNo',1,'ChannelNo',1,'Parameters',struct('DataFileSupport',struct('DataFileSelectedMaster',0,'DataFileSelectedLocal',0,'DataFileName','','DataFileDate','','SelectedFile',['<no file selected>']),'Options',struct('StatusSelected',1,'TimeSelected',1,'DeltaTimeSelected',1,'BytePortSelected',0,'MessageLengthSelected',0,'TriggerPort',struct('Selected',0,'TriggerType','rising'),'UserCoding',struct('Selected',0,'InterfaceFile','UserDecodingFile','FcnName','UserDecodeFcn','InportSelected',0,'InportWidth',1,'OutportSelected',0,'OutportWidth',1),'EnablePortSelected',0,'SignalOnPortnameSelected',1,'UseRXService',0),'Message',struct('MsgOnBlocknameSelected',0,'MsgName',['RX Message'],'MsgIdFormat',0,'MsgId',100,'MsgLength',8,'NumSignals',1,'SampleTime',-1,'Signal',struct('SgnName',['RX signal'],'SgnStartBit',0,'SgnLength',8,'SgnType',0,'ModeValue',-1,'DataType',0,'SLDataType','SS_DOUBLE','ByteLayout',0,'Factor',1,'Offset',0,'Min',0,'Max',255,'SgnComment',{{}},'SgnUnit',''),'MsgIdNumFormat',0,'MsgComment',{{''}}),'Version',1.2,'general',struct('isFromLib',1)),'GroupId',struct('Group',{{'RTICAN'}},'No',1,'Behavior',{{'NAMECHANGE'}},'BlockType',{{'SINK'}},'NameChangeFlag',0),'SFcnRTICANMessage',struct('MsgType','RX','MsgName',['RX Message'],'MsgIdFormat','STD','MsgId',100,'MsgLength',8,'NumSignals',1,'SampleTime',-1,'Signal',struct('SgnName',['RX signal'],'SgnStartBit',0,'SgnLength',8,'SgnType','standard','ModeValue',-1,'DataType',['unsigned int'],'ByteLayout',['little endian'],'SLDataType','SS_DOUBLE','Factor',1,'Offset',0),'StatusSelected','yes','TimeSelected','yes','DeltaTimeSelected','yes','BytePortSelected','no','MessageLengthSelected','no','EnablePortSelected','no','UserCoding',struct('Selected','no','InterfaceFile','UserDecodingFile','FcnName','UserDecodeFcn','InportSelected','no','InportWidth',1,'OutportSelected','no','OutportWidth',1),'TriggerPort',struct('Selected','no','TriggerType','rising'),'UseRXService','no','BoardType','DS4302','BoardNo',1,'ControllerNo',1,'SFcnPortType','Scalar'),'TLCFileName','rtican_rx_message')
      settings: AttributesFormatString=Group Id: RTICAN2\n
  Obstacle_Data_A_8_CAN : Outport
  wires:
  Bus Creator/1 -> Obstacle_Data_A_8_CAN/1
  Obstacle_Data_A_8/1 -> Bus Creator/1  "Alive_Counter_A_8"
  Obstacle_Data_A_8/2 -> Bus Creator/2  "ObjectIdentifier_A_8"
  Obstacle_Data_A_8/3 -> Bus Creator/3  "ObjectAge_A_8"
  Obstacle_Data_A_8/4 -> Bus Creator/4  "AngleRate_A_8"
  Obstacle_Data_A_8/5 -> Bus Creator/5  "AngleLeft_A_8"
  Obstacle_Data_A_8/6 -> Bus Creator/6  "AngleRight_A_8"
  Obstacle_Data_A_8/7 -> Bus Creator/7  "MotionStatus_A_8"
  Obstacle_Data_A_8/8 -> Bus Creator/8  "ObjectLane_A_8"
  Obstacle_Data_A_8/9 -> Bus Creator/9  "CIPV_A_8"
  Obstacle_Data_A_8/10 -> Bus Creator/10  "ObstacleBrakeLights_A_8"
  Obstacle_Data_A_8/11 -> Bus Creator/11  "BlinkerInfo_A_8"
